simulink model "sampleModel1667_5"  (R2023a)
settings: Solver=VariableStepAuto  StartTime=0.0  StopTime=10.0  RelTol=1e-3
libraries: hdlsllib x3, simulink x1
settings Model: Creator=user1  LastModifiedBy=user1

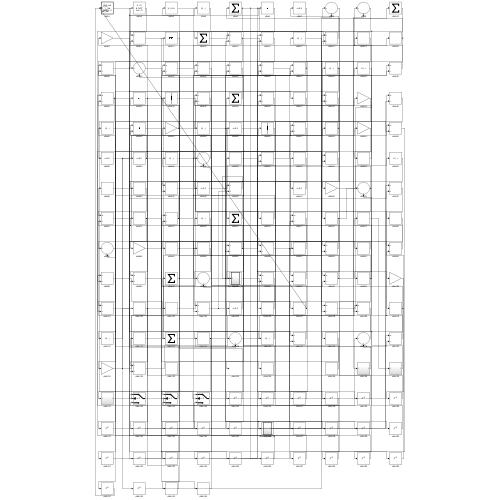
[thumbnail: Simulink's stored preview of the top-level diagram]
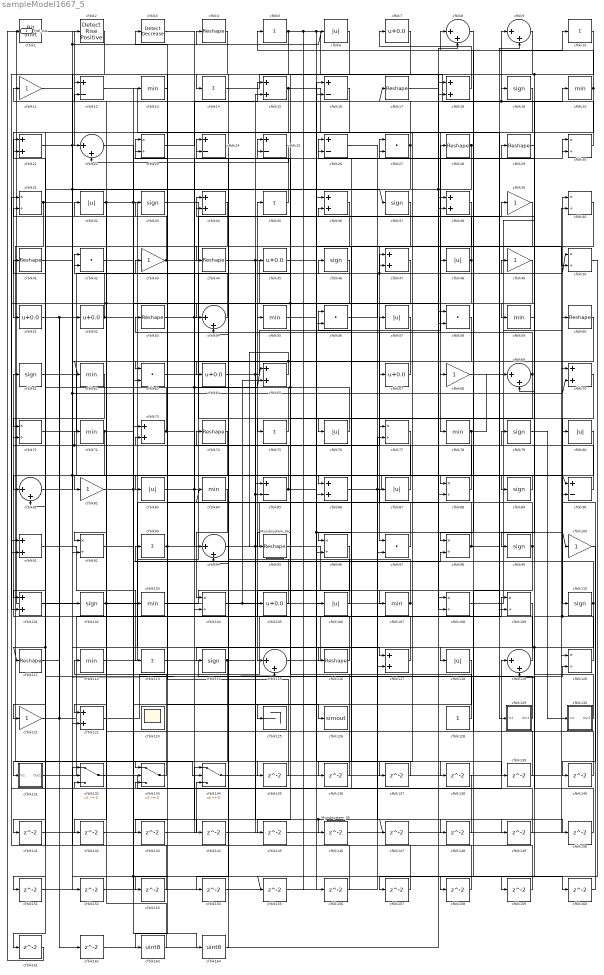
== system sampleModel1667_5 ==
  Mysubsystem_34 : Subsystem  TreatAsAtomicUnit=on  RTWFcnName=Mysubsystem_34
      settings: RTWFcnNameOpts=User specified  RTWFileNameOpts=Use function name
  Mysubsystem_35 : Subsystem  TreatAsAtomicUnit=on  RTWFcnName=Mysubsystem_35
      settings: RTWFcnNameOpts=User specified  RTWFileNameOpts=Use function name
  cfblk1 : hdlsllib/Logic and Bit Operations/Bit Shift  mode=Shift Left Logical  N=0
  cfblk{5,10,14,35,75,93,113} (7 alike) : Sum  Inputs=+  OutDataTypeStr=uint8
  cfblk{11,39,43,49,68,82,100,121} (8 alike) : Gain  OutDataTypeStr=uint8
  cfblk{15,18,21,34,36,38,47,65,70,73,86,91,101,117,122} (15 alike) : Sum  OutDataTypeStr=uint8
  cfblk{19,33,37,46,61,79,89,99,102,110,114} (11 alike) : Signum
  cfblk{13,20,55,59,62,72,78,84,103,107,112} (11 alike) : MinMax  OutDataTypeStr=uint8
  cfblk{23,30..31,40,50,71,77,88,92,96,98,104,108..109,120} (15 alike) : Product  Inputs=*/  OutDataTypeStr=uint8  RndMeth=Zero  SaturateOnIntegerOverflow=on
  cfblk{7,45,51..52,64,67,105} (7 alike) : Bias  Bias=0.0  SaturateOnIntegerOverflow=off
  cfblk{6,32,48,57,76,80,83,87,106,118} (10 alike) : Abs  OutDataTypeStr=uint8  SaturateOnIntegerOverflow=off
  cfblk{4,17,28..29,41,44,53,60,74,95,111,116} (12 alike) : Reshape
  cfblk{8..9,22,54,69,81,94,115,119} (9 alike) : Sum  Inputs=|++  OutDataTypeStr=uint8
  cfblk{12,16,24..26,85,90} (7 alike) : Sum  Inputs=+-  OutDataTypeStr=uint8
  cfblk123 : Scope
      settings: Floating=on
  cfblk125 : Terminator
  cfblk126 : ToWorkspace  VariableName=simout  SaveFormat=Timeseries  SampleTime=-1
  cfblk128 : Constant  OutDataTypeStr=uint8  SampleTime=-1
  cfblk129 : Subsystem
      settings: LibrarySourceBlock=|
      | hdlsllib/Ports &
      | Subsystems/Subsystem
  cfblk130 : Subsystem
      settings: LibrarySourceBlock=|
      | hdlsllib/Ports &
      | Subsystems/Subsystem
  cfblk131 : Subsystem
      settings: LibrarySourceBlock=|
      | hdlsllib/Ports &
      | Subsystems/Subsystem
  cfblk132 : Switch  OutDataTypeStr=uint8  SaturateOnIntegerOverflow=off  InputSameDT=off
  cfblk133 : Switch  OutDataTypeStr=uint8  SaturateOnIntegerOverflow=off  InputSameDT=off
  cfblk134 : Switch  OutDataTypeStr=uint8  SaturateOnIntegerOverflow=off  InputSameDT=off
  cfblk{135..162} (28 alike) : Delay  SampleTime=1
  cfblk163 : DataTypeConversion  OutDataTypeStr=uint8  SaturateOnIntegerOverflow=off  RndMeth=Floor
  cfblk164 : DataTypeConversion  OutDataTypeStr=uint8  SaturateOnIntegerOverflow=off  RndMeth=Floor
  cfblk2 : hdlsllib/Logic and Bit Operations/Detect Rise Positive  vinit=0  OutDataTypeStr=uint8
  cfblk{27,42,56,58,63,97} (6 alike) : DotProduct  OutDataTypeStr=uint8
  cfblk3 : simulink/Logic and Bit Operations/Detect Decrease  vinit=0.0  OutDataTypeStr=uint8
      settings: LibrarySourceBlock=|
      | hdlsllib/Logic and Bit
      | Operations/Detect
      | Decrease
  Hdl_out : Outport  OutDataTypeStr=uint8
  wires:
  cfblk32/1 -> cfblk117/1, cfblk58/2, cfblk122/1
  cfblk67/1 -> cfblk63/1
  cfblk43/1 -> cfblk39/1, cfblk21/2
  cfblk18/1 -> cfblk7/1
  cfblk111/1 -> cfblk102/1
  cfblk108/1 -> cfblk26/1
  cfblk97/1 -> cfblk23/1
  cfblk51/1 -> cfblk49/1, cfblk162/1
  cfblk93/1 -> cfblk43/1, cfblk30/1
  cfblk79/1 -> cfblk130/1(In1)
  cfblk2/1 -> cfblk22/1
  cfblk40/1 -> cfblk97/1
  cfblk4/1 -> cfblk14/1
  cfblk132/1 -> cfblk119/1
  cfblk13/1 -> cfblk83/1
  cfblk112/1 -> cfblk16/1
  cfblk121/1 -> cfblk35/1, cfblk52/1
  cfblk83/1 -> cfblk88/1, cfblk77/1
  cfblk14/1 -> cfblk20/1
  cfblk3/1 -> cfblk146/1, cfblk147/1
  cfblk103/1 -> cfblk107/1
  cfblk90/1 -> cfblk73/2
  cfblk1/1 -> cfblk12/1
  cfblk35/1 -> cfblk24/1
  cfblk12/1 -> cfblk78/1
  cfblk91/1 -> cfblk113/1
  cfblk53/1 -> cfblk76/1, cfblk67/1
  cfblk55/1 -> cfblk100/1, cfblk139/1
  cfblk31/1 -> cfblk134/2, cfblk160/1
  cfblk110/1 -> cfblk158/1, cfblk159/1, cfblk93/1
  cfblk88/1 -> cfblk55/1
  cfblk107/1 -> cfblk42/1, Hdl_out/1
  cfblk30/1 -> cfblk9/1, cfblk17/1
  cfblk37/1 -> cfblk86/1
  cfblk28/1 -> cfblk96/2, cfblk88/2, cfblk98/1
  cfblk65/1 -> Mysubsystem_34/1(In1), cfblk62/1
  cfblk86/1 -> cfblk89/1, cfblk138/1
  cfblk122/1 -> cfblk109/1
  cfblk85/1 -> cfblk21/1, cfblk72/1, cfblk36/1
  cfblk64/1 -> cfblk28/1, cfblk46/1
  cfblk16/1 -> cfblk51/1
  cfblk81/1 -> cfblk2/1, cfblk6/1, cfblk70/2
  cfblk87/1 -> cfblk57/1
  cfblk119/1 -> cfblk61/1
  cfblk23/1 -> cfblk15/1
  cfblk45/1 -> cfblk106/1
  cfblk94/1 -> cfblk47/2, cfblk50/1, cfblk18/1
  cfblk113/1 -> cfblk120/2
  cfblk27/1 -> cfblk11/1, cfblk81/1
  cfblk120/1 -> cfblk40/1, cfblk79/1
  cfblk92/1 -> cfblk98/2
  cfblk84/1 -> cfblk104/1
  cfblk70/1 -> cfblk110/1
  cfblk71/1 -> cfblk8/2
  cfblk56/1 -> cfblk48/1
  cfblk102/1 -> cfblk47/1, cfblk142/1
  cfblk33/1 -> cfblk80/1
  cfblk131/1(Out1) -> cfblk13/1
  cfblk129/1(Out1) -> cfblk41/1
  cfblk96/1 -> cfblk115/1
  cfblk8/1 -> cfblk68/1
  cfblk52/1 -> cfblk42/2, cfblk54/1
  cfblk46/1 -> cfblk101/1, cfblk92/1
  cfblk10/1 -> cfblk99/1, cfblk114/1
  cfblk17/1 -> cfblk108/1
  cfblk15/1 -> cfblk129/1(In1), cfblk81/2
  cfblk58/1 -> cfblk96/1
  cfblk41/1 -> cfblk115/2, cfblk90/1
  cfblk29/1 -> cfblk59/1
  cfblk44/1 -> cfblk108/2, cfblk30/2, cfblk149/1
  cfblk106/1 -> cfblk25/1
  cfblk115/1 -> cfblk9/2
  cfblk78/1 -> cfblk104/2, cfblk69/1
  cfblk6/1 -> cfblk101/2
  cfblk76/1 -> cfblk45/1, cfblk54/2
  cfblk63/1 -> cfblk75/1
  cfblk116/1 -> cfblk25/2
  cfblk69/1 -> cfblk53/1, cfblk125/1
  cfblk72/1 -> cfblk103/1, cfblk92/2
  cfblk20/1 -> cfblk86/2, cfblk5/1
  cfblk34/1 -> cfblk44/1
  cfblk133/1 -> cfblk112/1
  cfblk117/1 -> cfblk56/1
  cfblk57/1 -> cfblk63/2
  cfblk54/1 -> cfblk33/1
  cfblk89/1 -> cfblk82/1
  cfblk68/1 -> cfblk60/1
  cfblk5/1 -> cfblk38/2, cfblk50/2, cfblk156/1, cfblk122/2
  cfblk75/1 -> cfblk3/1
  cfblk73/1 -> cfblk65/1, cfblk27/1, cfblk31/2
  cfblk7/1 -> cfblk133/1
  cfblk128/1 -> cfblk105/1
  cfblk98/1 -> cfblk10/1, cfblk87/1
  cfblk36/1 -> cfblk71/1
  cfblk82/1 -> cfblk29/1, cfblk126/1
  cfblk21/1 -> cfblk4/1, cfblk116/1
  cfblk77/1 -> cfblk111/1, cfblk121/1
  cfblk42/1 -> cfblk155/1, cfblk164/1
  cfblk24/1 -> cfblk64/1
  cfblk38/1 -> cfblk131/1(In1)
  cfblk130/1(Out1) -> cfblk34/1
  cfblk99/1 -> cfblk118/1, cfblk69/2, cfblk34/2
  cfblk48/1 -> cfblk95/1, cfblk153/1, cfblk26/2
  cfblk105/1 -> cfblk84/1, cfblk24/2
  cfblk95/1 -> cfblk109/2
  cfblk25/1 -> cfblk22/2
  cfblk49/1 -> cfblk91/2
  cfblk59/1 -> cfblk19/1
  cfblk114/1 -> cfblk150/1, cfblk151/1
  cfblk11/1 -> cfblk117/2, cfblk37/1
  cfblk60/1 -> cfblk132/2
  cfblk104/1 -> cfblk85/2, cfblk27/2, cfblk65/2
  cfblk134/1 -> cfblk70/1
  cfblk61/1 -> cfblk94/1
  cfblk9/1 -> cfblk135/1
  cfblk135/1 -> cfblk23/2
  cfblk39/1 -> cfblk136/1
  cfblk136/1 -> cfblk85/1
  cfblk19/1 -> cfblk137/1
  cfblk137/1 -> cfblk133/2
  cfblk138/1 -> cfblk133/3
  cfblk139/1 -> cfblk12/2
  cfblk100/1 -> cfblk140/1
  cfblk140/1 -> cfblk8/1
  cfblk47/1 -> cfblk141/1
  cfblk141/1 -> cfblk134/1
  cfblk142/1 -> cfblk15/2
  cfblk118/1 -> cfblk143/1
  cfblk143/1 -> cfblk134/3
  cfblk22/1 -> cfblk144/1
  cfblk144/1 -> cfblk97/2
  cfblk80/1 -> cfblk145/1
  cfblk145/1 -> cfblk38/1
  cfblk146/1 -> cfblk120/1
  cfblk147/1 -> cfblk40/2
  cfblk26/1 -> cfblk148/1
  cfblk148/1 -> cfblk91/1
  cfblk149/1 -> cfblk36/2
  cfblk150/1 -> cfblk119/2
  cfblk151/1 -> cfblk77/2
  cfblk101/1 -> cfblk152/1
  cfblk152/1 -> cfblk73/1
  cfblk153/1 -> cfblk132/1
  cfblk109/1 -> cfblk154/1
  cfblk154/1 -> cfblk56/2
  cfblk155/1 -> cfblk16/2
  cfblk156/1 -> cfblk71/2
  cfblk50/1 -> cfblk157/1
  cfblk157/1 -> cfblk31/1
  cfblk158/1 -> cfblk132/3
  cfblk159/1 -> cfblk94/2
  cfblk160/1 -> cfblk90/2
  cfblk62/1 -> cfblk161/1
  cfblk161/1 -> cfblk1/1
  cfblk162/1 -> cfblk18/2
  cfblk74/1 -> cfblk163/1
  cfblk163/1 -> cfblk32/1
  cfblk164/1 -> cfblk74/1
  Mysubsystem_35/1(Out1) -> cfblk58/1

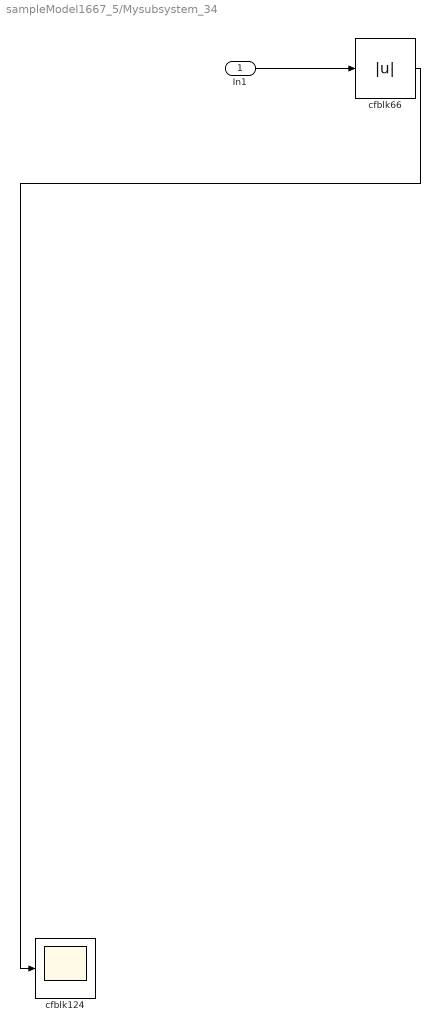
== system sampleModel1667_5/Mysubsystem_34 ==
  In1 : Inport
  cfblk124 : Scope
  cfblk66 : Abs  SaturateOnIntegerOverflow=off
  wires:
  cfblk66/1 -> cfblk124/1
  In1/1 -> cfblk66/1

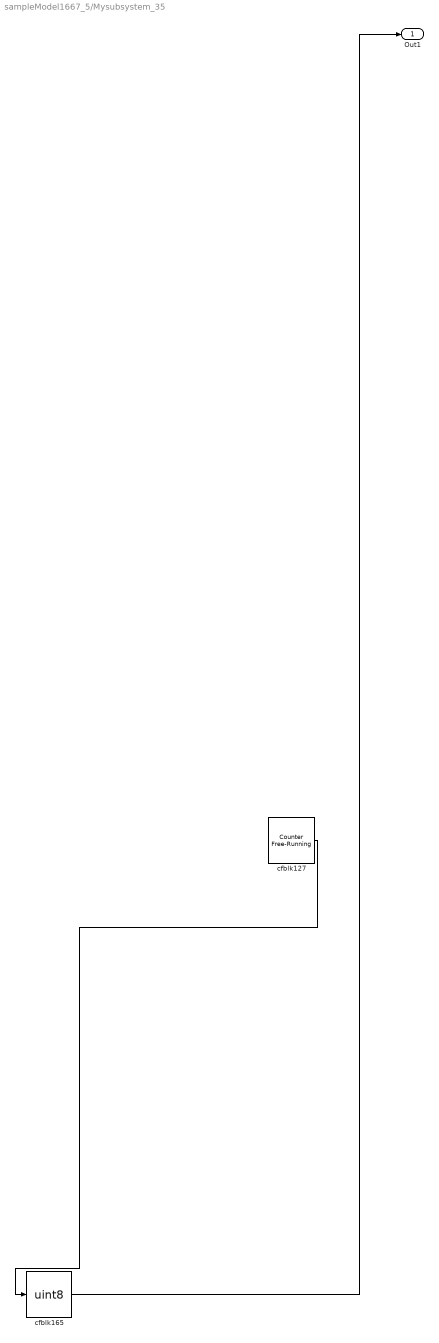
== system sampleModel1667_5/Mysubsystem_35 ==
  cfblk127 : hdlsllib/Sources/Counter Free-Running  NumBits=16  tsamp=-1
  cfblk165 : DataTypeConversion  OutDataTypeStr=uint8  SaturateOnIntegerOverflow=off  RndMeth=Floor
  Out1 : Outport
  wires:
  cfblk127/1 -> cfblk165/1
  cfblk165/1 -> Out1/1

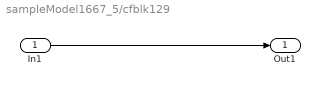
== system sampleModel1667_5/cfblk129 ==
  In1 : Inport
  Out1 : Outport
  wires:
  In1/1 -> Out1/1

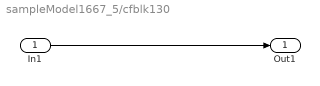
== system sampleModel1667_5/cfblk130 ==
  In1 : Inport
  Out1 : Outport
  wires:
  In1/1 -> Out1/1

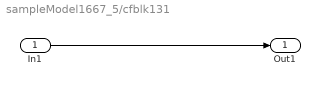
== system sampleModel1667_5/cfblk131 ==
  In1 : Inport
  Out1 : Outport
  wires:
  In1/1 -> Out1/1
